simulink model "SVPWMtrialsweird"  (R2015b)
settings: Solver=VariableStepAuto  StartTime=0.0  StopTime=0.05  RelTol=1e-3
libraries: powerlib x29, simulink x1
(part 2 of 2)

== matlab function SVPWMtrialsweird/sequencing ==
  data: a input; rgn2a input; rgn2b input; rgn3 input; rgn4 input; Sector1 input; Sector2 input; Sector3 input; Sector4 input; Sector5 input; Sector6 input; Ta input; Tb input; Tc input; Sa1 output; Sa2 output; Sa1P output; Sa2P output; time input; Sb1 output; Sb2 output; Sb1P output; Sb2P output; Sc1 output; Sc2 output; Sc1P output; Sc2P output; exttime input
function [Sa1, Sa2, Sa1P, Sa2P, Sb1, Sb2, Sb1P, Sb2P, Sc1, Sc2, Sc1P, Sc2P] = fcn(a,rgn2a,rgn2b,rgn3,rgn4,Sector1,Sector2, Sector3, Sector4, Sector5,Sector6,Ta, Tb, Tc, time,exttime)
% this program works for magnitude of Vref is greater then Vd/3 meaning ma
% must be greater than 1/sqrt(3). for smaller ma's computation is a bit
% more tricky therefore it is omitted for simplicity for now. 
% % Vref = ma*Vd/sqrt(3); %magnitude of Vref
% % theta = 2*pi*fundf*time; %angle of Vref
% % angle = mod(theta, 2*pi);
% % Ts = 1/swf;
% % Ta = 0;
% % Tb = 0;
% % Tc = 0;
% % output = 0;
% % Sector1 = 0; Sector2 = 0; Sector3 = 0; Sector4= 0; Sector5 = 0; Sector6 = 0;
% % rgn2 = 0 ; rgn3 = 0; rgn4 = 0;
Sa1=0; Sa2=0; Sa1P=0; Sa2P=0; Sb1=0; Sb2=0; Sb1P=0; Sb2P=0; Sc1=0; Sc2=0; Sc1P=0; Sc2P=0;
%a = exttime;
%% Sequencing Part
if(Sector1)
    if(rgn3)
        while(a<exttime+Tc/4)
            Sa1=0; Sa2=1; Sa1P=1; Sa2P=0;
            Sb1=0; Sb2=0; Sb1P=1; Sb2P=1; 
            Sc1=0; Sc2=0; Sc1P=1; Sc2P=1;
            a = a+0.000001; %pause(Tc/4); 
        end
        while(a<exttime+Tb/2)
            Sa1=1; Sa2=1; Sa1P=0; Sa2P=0;
            Sb1=0; Sb2=0; Sb1P=1; Sb2P=1; 
            Sc1=0; Sc2=0; Sc1P=1; Sc2P=1;
            a = a+0.000001;%pause(Tb/2);
        end
        while(a<exttime+Ta/2)
            Sa1=1; Sa2=1; Sa1P=0; Sa2P=0;
            Sb1=0; Sb2=1; Sb1P=1; Sb2P=0; 
            Sc1=0; Sc2=0; Sc1P=1; Sc2P=1;
            a = a+0.000001; %pause(Ta/2); 
        end
        while(a<exttime+Tc/2)
            Sa1=1; Sa2=1; Sa1P=0; Sa2P=0;
            Sb1=0; Sb2=1; Sb1P=1; Sb2P=0; 
            Sc1=0; Sc2=1; Sc1P=1; Sc2P=0;
            a = a+0.000001; %pause(Tc/2);
        end
        while(a<exttime+Ta/2)
            Sa1=1; Sa2=1; Sa1P=0; Sa2P=0;
            Sb1=0; Sb2=1; Sb1P=1; Sb2P=0; 
            Sc1=0; Sc2=0; Sc1P=1; Sc2P=1;
            a = a+0.000001; %pause(Ta/2); 
        end
        while(a<exttime+Tb/2)
            Sa1=1; Sa2=1; Sa1P=0; Sa2P=0;
            Sb1=0; Sb2=0; Sb1P=1; Sb2P=1; 
            Sc1=0; Sc2=0; Sc1P=1; Sc2P=1;
            a = a+0.000001; %pause(Tb/2); 
        end
        while(a<exttime+Tc/4)
            Sa1=0; Sa2=1; Sa1P=1; Sa2P=0;
            Sb1=0; Sb2=0; Sb1P=1; Sb2P=1; 
            Sc1=0; Sc2=0; Sc1P=1; Sc2P=1;
            a = a+0.000001; %pause(Tc/4);        
        end
    end

        if(rgn2a)
            while(a<exttime+Tc/4)
                Sa1=0; Sa2=1; Sa1P=1; Sa2P=0;
                Sb1=0; Sb2=0; Sb1P=1; Sb2P=1; 
                Sc1=0; Sc2=0; Sc1P=1; Sc2P=1;
            a = a+0.000001; %pause(Tc/4);
            end
            while(a<exttime+Tb/2)
                Sa1=0; Sa2=1; Sa1P=1; Sa2P=0;
                Sb1=0; Sb2=1; Sb1P=1; Sb2P=0; 
                Sc1=0; Sc2=0; Sc1P=1; Sc2P=1;
                a = a+0.000001; %pause(Tb/2); 
            end
            while(a<exttime+Ta/2)
                Sa1=1; Sa2=1; Sa1P=0; Sa2P=0;
                Sb1=0; Sb2=1; Sb1P=1; Sb2P=0; 
                Sc1=0; Sc2=0; Sc1P=1; Sc2P=1;       
                a = a+0.000001; %pause(Ta/2); 
            end
            while(a<exttime+Tc/2)
                Sa1=1; Sa2=1; Sa1P=0; Sa2P=0;
                Sb1=0; Sb2=1; Sb1P=1; Sb2P=0; 
                Sc1=0; Sc2=1; Sc1P=1; Sc2P=0;
            a = a+0.000001; %pause(Tc/2);
            end
            while(a<exttime+Ta/2)
                Sa1=1; Sa2=1; Sa1P=0; Sa2P=0;
                Sb1=0; Sb2=1; Sb1P=1; Sb2P=0; 
                Sc1=0; Sc2=0; Sc1P=1; Sc2P=1;
                a = a+0.000001; %pause(Ta/2); 
            end
            while(a<exttime+Tb/2)
                Sa1=0; Sa2=1; Sa1P=1; Sa2P=0;
                Sb1=0; Sb2=1; Sb1P=1; Sb2P=0; 
                Sc1=0; Sc2=0; Sc1P=1; Sc2P=1;
                a = a+0.000001; %pause(Tb/2); 
            end
            while(a<exttime+Tc/4)
                Sa1=0; Sa2=1; Sa1P=1; Sa2P=0;
                Sb1=0; Sb2=0; Sb1P=1; Sb2P=1; 
                Sc1=0; Sc2=0; Sc1P=1; Sc2P=1;
                a = a+0.000001; %pause(Tc/4);        
            end
        end
        if(rgn2b)
            while(a<exttime+Tc/4)
                Sa1=0; Sa2=1; Sa1P=1; Sa2P=0;
                Sb1=0; Sb2=1; Sb1P=1; Sb2P=0; 
                Sc1=0; Sc2=0; Sc1P=1; Sc2P=1;
                a = a+0.000001; %pause(Tc/4);
            end
            while(a<exttime+Tb/2)
                Sa1=1; Sa2=1; Sa1P=0; Sa2P=0;
                Sb1=0; Sb2=1; Sb1P=1; Sb2P=0; 
                Sc1=0; Sc2=0; Sc1P=1; Sc2P=1;
                a = a+0.000001; %pause(Tb/2); 
            end
            while(a<exttime+Ta/2)
                Sa1=1; Sa2=1; Sa1P=0; Sa2P=0;
                Sb1=0; Sb2=1; Sb1P=1; Sb2P=0; 
                Sc1=0; Sc2=1; Sc1P=1; Sc2P=0;
                a = a+0.000001; %pause(Ta/2); 
            end
            while(a<exttime+Tc/2)
                Sa1=1; Sa2=1; Sa1P=0; Sa2P=0;
                Sb1=1; Sb2=1; Sb1P=0; Sb2P=0; 
                Sc1=0; Sc2=1; Sc1P=1; Sc2P=0;
                a = a+0.000001; %pause(Tc/2);
            end
            while(a<exttime+Ta/2)
                Sa1=1; Sa2=1; Sa1P=0; Sa2P=0;
                Sb1=0; Sb2=1; Sb1P=1; Sb2P=0; 
                Sc1=0; Sc2=1; Sc1P=1; Sc2P=0;
                a = a+0.000001; %pause(Ta/2); 
            end
            while(a<exttime+Tb/2)
                Sa1=1; Sa2=1; Sa1P=0; Sa2P=0;
                Sb1=0; Sb2=1; Sb1P=1; Sb2P=0; 
                Sc1=0; Sc2=0; Sc1P=1; Sc2P=1;
                a = a+0.000001; %pause(Tb/2); 
            end
            while(a<exttime+Tc/4)
                Sa1=0; Sa2=1; Sa1P=1; Sa2P=0;
                Sb1=0; Sb2=1; Sb1P=1; Sb2P=0; 
                Sc1=0; Sc2=0; Sc1P=1; Sc2P=1;
                a = a+0.000001; %pause(Tc/4);
            end
        end
    if(rgn4)
        while(a<exttime+Tc/4)
            Sa1=0; Sa2=1; Sa1P=1; Sa2P=0;
            Sb1=0; Sb2=1; Sb1P=1; Sb2P=0;
            Sc1=0; Sc2=0; Sc1P=1; Sc2P=1;
            a = a+0.000001; %pause(Tc/4);
        end
        while(a<exttime+Tb/2)
            Sa1=1; Sa2=1; Sa1P=0; Sa2P=0;
            Sb1=0; Sb2=1; Sb1P=1; Sb2P=0;
            Sc1=0; Sc2=0; Sc1P=1; Sc2P=1;        
            a = a+0.000001; %pause(Tb/2);         
        end
        while(a<exttime+Ta/2)
            Sa1=1; Sa2=1; Sa1P=0; Sa2P=0;
            Sb1=1; Sb2=1; Sb1P=0; Sb2P=0;
            Sc1=0; Sc2=0; Sc1P=1; Sc2P=1;
            a = a+0.000001; %pause(Ta/2); 
        end
        while(a<exttime+Tc/2)
            Sa1=1; Sa2=1; Sa1P=0; Sa2P=0;
            Sb1=1; Sb2=1; Sb1P=0; Sb2P=0;
            Sc1=0; Sc2=1; Sc1P=1; Sc2P=0;
            a = a+0.000001; %pause(Tc/2);
        end
        while(a<exttime+Ta/2)
            Sa1=1; Sa2=1; Sa1P=0; Sa2P=0;
            Sb1=1; Sb2=1; Sb1P=0; Sb2P=0;
            Sc1=0; Sc2=0; Sc1P=1; Sc2P=1;
            a = a+0.000001; %pause(Ta/2);         
        end
        while(a<exttime+Tb/2)
            Sa1=1; Sa2=1; Sa1P=0; Sa2P=0;
            Sb1=0; Sb2=1; Sb1P=1; Sb2P=0;
            Sc1=0; Sc2=0; Sc1P=1; Sc2P=1;        
            a = a+0.000001; %pause(Tb/2); 
        end
        while(a<exttime+Tc/4)
            Sa1=0; Sa2=1; Sa1P=1; Sa2P=0;
            Sb1=0; Sb2=1; Sb1P=1; Sb2P=0;
            Sc1=0; Sc2=0; Sc1P=1; Sc2P=1;
            a = a+0.000001; %pause(Tc/4);
        end
    end
end
if(Sector2)
    if(rgn3)
        while(a<exttime+Tc/4)
            Sa1=0; Sa2=1; Sa1P=1; Sa2P=0;
            Sb1=0; Sb2=1; Sb1P=1; Sb2P=0;
            Sc1=0; Sc2=0; Sc1P=1; Sc2P=1;
        a = a+0.000001; %pause(Tc/4);
        end
        while(a<exttime+Tb/2)
            Sa1=0; Sa2=1; Sa1P=1; Sa2P=0;
            Sb1=1; Sb2=1; Sb1P=0; Sb2P=0;
            Sc1=0; Sc2=0; Sc1P=1; Sc2P=1;
            a = a+0.000001; %pause(Tb/2); 
        end
        while(a<exttime+Ta/2)
            Sa1=1; Sa2=1; Sa1P=0; Sa2P=0;
            Sb1=1; Sb2=1; Sb1P=0; Sb2P=0;
            Sc1=0; Sc2=0; Sc1P=1; Sc2P=1;
            a = a+0.000001; %pause(Ta/2); 
        end
        while(a<exttime+Tc/2)
            Sa1=1; Sa2=1; Sa1P=0; Sa2P=0;
            Sb1=1; Sb2=1; Sb1P=0; Sb2P=0;
            Sc1=0; Sc2=1; Sc1P=1; Sc2P=0;       
            a = a+0.000001; %pause(Tc/2);
        end
        while(a<exttime+Ta/2)
            Sa1=1; Sa2=1; Sa1P=0; Sa2P=0;
            Sb1=1; Sb2=1; Sb1P=0; Sb2P=0;
            Sc1=0; Sc2=0; Sc1P=1; Sc2P=1;
            a = a+0.000001; %pause(Ta/2); 
        end
        while(a<exttime+Tb/2)
            Sa1=0; Sa2=1; Sa1P=1; Sa2P=0;
            Sb1=1; Sb2=1; Sb1P=0; Sb2P=0;
            Sc1=0; Sc2=0; Sc1P=1; Sc2P=1;
            a = a+0.000001; %pause(Tb/2); 
        end
        while(a<exttime+Tc/4)
            Sa1=0; Sa2=1; Sa1P=1; Sa2P=0;
            Sb1=0; Sb2=1; Sb1P=1; Sb2P=0;
            Sc1=0; Sc2=0; Sc1P=1; Sc2P=1;
            a = a+0.000001; %pause(Tc/4);       
        end
    end
    
        if(rgn2a)
            while(a<exttime+Tc/4)
                Sa1=0; Sa2=1; Sa1P=1; Sa2P=0;
                Sb1=0; Sb2=1; Sb1P=1; Sb2P=0;
                Sc1=0; Sc2=0; Sc1P=1; Sc2P=1;
                a = a+0.000001; %pause(Tc/4);
            end
            while(a<exttime+Tb/2)
                Sa1=0; Sa2=1; Sa1P=1; Sa2P=0;
                Sb1=1; Sb2=1; Sb1P=0; Sb2P=0;
                Sc1=0; Sc2=0; Sc1P=1; Sc2P=1;
                a = a+0.000001; %pause(Tb/2); 
            end
            while(a<exttime+Ta/2)
                Sa1=0; Sa2=1; Sa1P=1; Sa2P=0;
                Sb1=1; Sb2=1; Sb1P=0; Sb2P=0;
                Sc1=0; Sc2=1; Sc1P=1; Sc2P=0;
                a = a+0.000001; %pause(Ta/2); 
            end
            while(a<exttime+Tc/2)
                Sa1=1; Sa2=1; Sa1P=0; Sa2P=0;
                Sb1=1; Sb2=1; Sb1P=0; Sb2P=0;
                Sc1=0; Sc2=1; Sc1P=1; Sc2P=0;            
                a = a+0.000001; %pause(Tc/2);
            end
            while(a<exttime+Ta/2)
                Sa1=0; Sa2=1; Sa1P=1; Sa2P=0;
                Sb1=1; Sb2=1; Sb1P=0; Sb2P=0;
                Sc1=0; Sc2=1; Sc1P=1; Sc2P=0;
                a = a+0.000001; %pause(Ta/2); 
            end
            while(a<exttime+Tb/2)
                Sa1=0; Sa2=1; Sa1P=1; Sa2P=0;
                Sb1=1; Sb2=1; Sb1P=0; Sb2P=0;
                Sc1=0; Sc2=0; Sc1P=1; Sc2P=1;
                a = a+0.000001; %pause(Tb/2); 
            end
            while(a<exttime+Tc/4)
                Sa1=0; Sa2=1; Sa1P=1; Sa2P=0;
                Sb1=0; Sb2=1; Sb1P=1; Sb2P=0;
                Sc1=0; Sc2=0; Sc1P=1; Sc2P=1;
                a = a+0.000001; %pause(Tc/4);
            end
        end
        if(rgn2b)
            while(a<exttime+Tc/4)
                Sa1=0; Sa2=0; Sa1P=1; Sa2P=1;
                Sb1=0; Sb2=1; Sb1P=1; Sb2P=0;
                Sc1=0; Sc2=0; Sc1P=1; Sc2P=1;
                a = a+0.000001; %pause(Tc/4);
            end
            while(a<exttime+Tb/2)
                Sa1=0; Sa2=1; Sa1P=1; Sa2P=0;
                Sb1=0; Sb2=1; Sb1P=1; Sb2P=0;
                Sc1=0; Sc2=0; Sc1P=1; Sc2P=1;
                a = a+0.000001; %pause(Tb/2); 
            end
            while(a<exttime+Ta/2)
                Sa1=0; Sa2=1; Sa1P=1; Sa2P=0;
                Sb1=1; Sb2=1; Sb1P=0; Sb2P=0;
                Sc1=0; Sc2=0; Sc1P=1; Sc2P=1;
                a = a+0.000001; %pause(Ta/2); 
            end
            while(a<exttime+Tc/2)
                Sa1=0; Sa2=1; Sa1P=1; Sa2P=0;   
                Sb1=1; Sb2=1; Sb1P=0; Sb2P=0;
                Sc1=0; Sc2=1; Sc1P=1; Sc2P=0;
                a = a+0.000001; %pause(Tc/2);
            end
            while(a<exttime+Ta/2)
                Sa1=0; Sa2=1; Sa1P=1; Sa2P=0;
                Sb1=1; Sb2=1; Sb1P=0; Sb2P=0;
                Sc1=0; Sc2=0; Sc1P=1; Sc2P=1;
                a = a+0.000001; %pause(Ta/2); 
            end
            while(a<exttime+Tb/2)
                Sa1=0; Sa2=1; Sa1P=1; Sa2P=0;
                Sb1=0; Sb2=1; Sb1P=1; Sb2P=0;
                Sc1=0; Sc2=0; Sc1P=1; Sc2P=1;
                a = a+0.000001; %pause(Tb/2); 
            end
            while(a<exttime+Tc/4)
                Sa1=0; Sa2=0; Sa1P=1; Sa2P=1;
                Sb1=0; Sb2=1; Sb1P=1; Sb2P=0;
                Sc1=0; Sc2=0; Sc1P=1; Sc2P=1;
                a = a+0.000001; %pause(Tc/4);           
            end
        end    
    if(rgn4)
        while(a<exttime+Tc/4)
            Sa1=0; Sa2=0; Sa1P=1; Sa2P=1;
            Sb1=0; Sb2=1; Sb1P=1; Sb2P=0;
            Sc1=0; Sc2=0; Sc1P=1; Sc2P=1;
            a = a+0.000001; %pause(Tc/4);
        end
        while(a<exttime+Tb/2)
            Sa1=0; Sa2=0; Sa1P=1; Sa2P=1;
            Sb1=1; Sb2=1; Sb1P=0; Sb2P=0;
            Sc1=0; Sc2=0; Sc1P=1; Sc2P=1;
            a = a+0.000001; %pause(Tb/2); 
        end
        while(a<exttime+Ta/2)
            Sa1=0; Sa2=1; Sa1P=1; Sa2P=0;
            Sb1=1; Sb2=1; Sb1P=0; Sb2P=0;
            Sc1=0; Sc2=0; Sc1P=1; Sc2P=1;
            a = a+0.000001; %pause(Ta/2); 
        end
        while(a<exttime+Tc/2)
            Sa1=0; Sa2=1; Sa1P=1; Sa2P=0;
            Sb1=1; Sb2=1; Sb1P=0; Sb2P=0;
            Sc1=0; Sc2=1; Sc1P=1; Sc2P=0;
            a = a+0.000001; %pause(Tc/2); 
        end
        while(a<exttime+Ta/2)
            Sa1=0; Sa2=1; Sa1P=1; Sa2P=0;
            Sb1=1; Sb2=1; Sb1P=0; Sb2P=0;
            Sc1=0; Sc2=0; Sc1P=1; Sc2P=1;
            a = a+0.000001; %pause(Ta/2); 
        end
        while(a<exttime+Tb/2)
            Sa1=0; Sa2=0; Sa1P=1; Sa2P=1;
            Sb1=1; Sb2=1; Sb1P=0; Sb2P=0;
            Sc1=0; Sc2=0; Sc1P=1; Sc2P=1;
            a = a+0.000001; %pause(Tb/2); 
        end
        while(a<exttime+Tc/4)
            Sa1=0; Sa2=0; Sa1P=1; Sa2P=1;
            Sb1=0; Sb2=1; Sb1P=1; Sb2P=0;
            Sc1=0; Sc2=0; Sc1P=1; Sc2P=1;
            a = a+0.000001; %pause(Tc/4);
        end
    end

end
if(Sector3)
    if(rgn3)
        while(a<exttime+Tc/4)
            Sa1=0; Sa2=0; Sa1P=1; Sa2P=1;
            Sb1=0; Sb2=1; Sb1P=1; Sb2P=0;
            Sc1=0; Sc2=0; Sc1P=1; Sc2P=1;
            a = a+0.000001; %pause(Tc/4);
        end
        while(a<exttime+Tb/2)
            Sa1=0; Sa2=0; Sa1P=1; Sa2P=1;
            Sb1=1; Sb2=1; Sb1P=0; Sb2P=0;
            Sc1=0; Sc2=0; Sc1P=1; Sc2P=1;
            a = a+0.000001; %pause(Tb/2); 
        end
        while(a<exttime+Ta/2)
            Sa1=0; Sa2=0; Sa1P=1; Sa2P=1;
            Sb1=1; Sb2=1; Sb1P=0; Sb2P=0;
            Sc1=0; Sc2=1; Sc1P=1; Sc2P=0;
            a = a+0.000001; %pause(Ta/2); 
        end
        while(a<exttime+Tc/2)
            Sa1=0; Sa2=1; Sa1P=1; Sa2P=0;
            Sb1=1; Sb2=1; Sb1P=0; Sb2P=0;
            Sc1=0; Sc2=1; Sc1P=1; Sc2P=0;
            a = a+0.000001; %pause(Tc/2);
        end
        while(a<exttime+Ta/2)
            Sa1=0; Sa2=0; Sa1P=1; Sa2P=1;
            Sb1=1; Sb2=1; Sb1P=0; Sb2P=0;
            Sc1=0; Sc2=1; Sc1P=1; Sc2P=0;
            a = a+0.000001; %pause(Ta/2); 
        end
        while(a<exttime+Tb/2)
            Sa1=0; Sa2=0; Sa1P=1; Sa2P=1;
            Sb1=1; Sb2=1; Sb1P=0; Sb2P=0;
            Sc1=0; Sc2=0; Sc1P=1; Sc2P=1;
            a = a+0.000001; %pause(Tb/2); 
        end
        while(a<exttime+Tc/4)
            Sa1=0; Sa2=0; Sa1P=1; Sa2P=1;
            Sb1=0; Sb2=1; Sb1P=1; Sb2P=0;
            Sc1=0; Sc2=0; Sc1P=1; Sc2P=1;
            a = a+0.000001; %pause(Tc/4);        
        end
    end

        if(rgn2a)
            while(a<exttime+Tc/4)            
                Sa1=0; Sa2=0; Sa1P=1; Sa2P=1;
                Sb1=0; Sb2=1; Sb1P=1; Sb2P=0;
                Sc1=0; Sc2=0; Sc1P=1; Sc2P=1;
                a = a+0.000001; %pause(Tc/4);
            end
            while(a<exttime+Tb/2)
                Sa1=0; Sa2=0; Sa1P=1; Sa2P=1;
                Sb1=0; Sb2=1; Sb1P=1; Sb2P=0;
                Sc1=0; Sc2=1; Sc1P=1; Sc2P=0;
                a = a+0.000001; %pause(Tb/2); 
            end
            while(a<exttime+Ta/2)
                Sa1=0; Sa2=0; Sa1P=1; Sa2P=1;
                Sb1=1; Sb2=1; Sb1P=0; Sb2P=0;
                Sc1=0; Sc2=1; Sc1P=1; Sc2P=0;
            	a = a+0.000001; %pause(Ta/2); 
            end
            while(a<exttime+Tc/2)
                Sa1=0; Sa2=0; Sa1P=1; Sa2P=1;
                Sb1=1; Sb2=1; Sb1P=0; Sb2P=0;
                Sc1=0; Sc2=0; Sc1P=1; Sc2P=1;
                a = a+0.000001; %pause(Tc/2);
            end
            while(a<exttime+Ta/2)
                Sa1=0; Sa2=0; Sa1P=1; Sa2P=1;
                Sb1=1; Sb2=1; Sb1P=0; Sb2P=0;
                Sc1=0; Sc2=1; Sc1P=1; Sc2P=0;
                a = a+0.000001; %pause(Ta/2); 
            end
            while(a<exttime+Tb/2)
                Sa1=0; Sa2=0; Sa1P=1; Sa2P=1;
                Sb1=0; Sb2=1; Sb1P=1; Sb2P=0;
                Sc1=0; Sc2=1; Sc1P=1; Sc2P=0;
                a = a+0.000001; %pause(Tb/2); 
            end
            while(a<exttime+Tc/4)
                Sa1=0; Sa2=0; Sa1P=1; Sa2P=1;
                Sb1=0; Sb2=1; Sb1P=1; Sb2P=0;
                Sc1=0; Sc2=0; Sc1P=1; Sc2P=1;
                a = a+0.000001; %pause(Tc/4); 
            end
        end
        if(rgn2b)
            while(a<exttime+Tc/4)
                Sa1=0; Sa2=0; Sa1P=1; Sa2P=1;
                Sb1=0; Sb2=1; Sb1P=1; Sb2P=0;
                Sc1=0; Sc2=1; Sc1P=1; Sc2P=0;
                a = a+0.000001; %pause(Tc/4);
            end
            while(a<exttime+Tb/2)
                Sa1=0; Sa2=0; Sa1P=1; Sa2P=1;
                Sb1=1; Sb2=1; Sb1P=0; Sb2P=0;
                Sc1=0; Sc2=1; Sc1P=1; Sc2P=0;
                a = a+0.000001; %pause(Tb/2); 
            end
            while(a<exttime+Ta/2)
                Sa1=0; Sa2=1; Sa1P=1; Sa2P=0;
                Sb1=1; Sb2=1; Sb1P=0; Sb2P=0;
                Sc1=0; Sc2=1; Sc1P=1; Sc2P=0;
                a = a+0.000001; %pause(Ta/2); 
            end
            while(a<exttime+Tc/2)
                Sa1=0; Sa2=1; Sa1P=1; Sa2P=0;
                Sb1=1; Sb2=1; Sb1P=0; Sb2P=0;
                Sc1=1; Sc2=1; Sc1P=0; Sc2P=0;
                a = a+0.000001; %pause(Tc/2);
            end
            while(a<exttime+Ta/2)
                Sa1=0; Sa2=1; Sa1P=1; Sa2P=0;
                Sb1=1; Sb2=1; Sb1P=0; Sb2P=0;
                Sc1=0; Sc2=1; Sc1P=1; Sc2P=0;
                a = a+0.000001; %pause(Ta/2); 
            end
            while(a<exttime+Tb/2)
                Sa1=0; Sa2=0; Sa1P=1; Sa2P=1;
                Sb1=1; Sb2=1; Sb1P=0; Sb2P=0;
                Sc1=0; Sc2=1; Sc1P=1; Sc2P=0;
                a = a+0.000001; %pause(Tb/2); 
            end
            while(a<exttime+Tc/4)
                Sa1=0; Sa2=0; Sa1P=1; Sa2P=1;
                Sb1=0; Sb2=1; Sb1P=1; Sb2P=0;
                Sc1=0; Sc2=1; Sc1P=1; Sc2P=0;
                a = a+0.000001; %pause(Tc/4);            
            end
        end

    if(rgn4)
        while(a<exttime+Tc/4)
            Sa1=0; Sa2=0; Sa1P=1; Sa2P=1;
            Sb1=0; Sb2=1; Sb1P=1; Sb2P=0;
            Sc1=0; Sc2=1; Sc1P=1; Sc2P=0;
            a = a+0.000001; %pause(Tc/4);
        end
        while(a<exttime+Tb/2)
            Sa1=0; Sa2=0; Sa1P=1; Sa2P=1;
            Sb1=1; Sb2=1; Sb1P=0; Sb2P=0;
            Sc1=0; Sc2=1; Sc1P=1; Sc2P=0;
            a = a+0.000001; %pause(Tb/2); 
        end
        while(a<exttime+Ta/2)
            Sa1=0; Sa2=0; Sa1P=1; Sa2P=1;
            Sb1=1; Sb2=1; Sb1P=0; Sb2P=0;
            Sc1=1; Sc2=1; Sc1P=0; Sc2P=0;
            a = a+0.000001; %pause(Ta/2); 
        end
        while(a<exttime+Tc/2)
            Sa1=0; Sa2=1; Sa1P=1; Sa2P=0;
            Sb1=1; Sb2=1; Sb1P=0; Sb2P=0;
            Sc1=1; Sc2=1; Sc1P=0; Sc2P=0;
            a = a+0.000001; %pause(Tc/2);
        end
        while(a<exttime+Ta/2)
            Sa1=0; Sa2=0; Sa1P=1; Sa2P=1;
            Sb1=1; Sb2=1; Sb1P=0; Sb2P=0;
            Sc1=1; Sc2=1; Sc1P=0; Sc2P=0;
            a = a+0.000001; %pause(Ta/2); 
        end
        while(a<exttime+Tb/2)
            Sa1=0; Sa2=0; Sa1P=1; Sa2P=1;
            Sb1=1; Sb2=1; Sb1P=0; Sb2P=0;
            Sc1=0; Sc2=1; Sc1P=1; Sc2P=0;
            a = a+0.000001; %pause(Tb/2); 
        end
        while(a<exttime+Tc/4)
            Sa1=0; Sa2=0; Sa1P=1; Sa2P=1;
            Sb1=0; Sb2=1; Sb1P=1; Sb2P=0;
            Sc1=0; Sc2=1; Sc1P=1; Sc2P=0;
            a = a+0.000001; %pause(Tc/4);
        end
    end
end
if(Sector4)
    if(rgn3) 
        while(a<exttime+Tc/4)
            Sa1=0; Sa2=1; Sa1P=1; Sa2P=0;
            Sb1=1; Sb2=1; Sb1P=0; Sb2P=0;
            Sc1=1; Sc2=1; Sc1P=0; Sc2P=0;
            a = a+0.000001; %pause(Tc/4);
        end
        while(a<exttime+Tb/2)
            Sa1=0; Sa2=0; Sa1P=1; Sa2P=1;
            Sb1=1; Sb2=1; Sb1P=0; Sb2P=0;
            Sc1=1; Sc2=1; Sc1P=0; Sc2P=0;
            a = a+0.000001; %pause(Tb/2); 
        end
        while(a<exttime+Ta/2)
            Sa1=0; Sa2=0; Sa1P=1; Sa2P=1;
            Sb1=0; Sb2=1; Sb1P=1; Sb2P=0;
            Sc1=1; Sc2=1; Sc1P=0; Sc2P=0;
            a = a+0.000001; %pause(Ta/2); 
        end
        while(a<exttime+Tc/2)
            Sa1=0; Sa2=0; Sa1P=1; Sa2P=1;
            Sb1=0; Sb2=1; Sb1P=1; Sb2P=0;
            Sc1=0; Sc2=1; Sc1P=1; Sc2P=0;
            a = a+0.000001; %pause(Tc/2);
        end
        while(a<exttime+Ta/2)
            Sa1=0; Sa2=0; Sa1P=1; Sa2P=1;
            Sb1=0; Sb2=1; Sb1P=1; Sb2P=0;
            Sc1=1; Sc2=1; Sc1P=0; Sc2P=0;
            a = a+0.000001; %pause(Ta/2); 
        end
        while(a<exttime+Tb/2)
            Sa1=0; Sa2=0; Sa1P=1; Sa2P=1;
            Sb1=1; Sb2=1; Sb1P=0; Sb2P=0;
            Sc1=1; Sc2=1; Sc1P=0; Sc2P=0;
            a = a+0.000001; %pause(Tb/2); 
        end
        while(a<exttime+Tc/4)
            Sa1=0; Sa2=1; Sa1P=1; Sa2P=0;
            Sb1=1; Sb2=1; Sb1P=0; Sb2P=0;
            Sc1=1; Sc2=1; Sc1P=0; Sc2P=0;
            a = a+0.000001; %pause(Tc/4);
        end
    end
        if(rgn2a)
            while(a<exttime+Tc/4)
                Sa1=0; Sa2=1; Sa1P=1; Sa2P=0;
                Sb1=1; Sb2=1; Sb1P=0; Sb2P=0;
                Sc1=1; Sc2=1; Sc1P=0; Sc2P=0;
                a = a+0.000001; %pause(Tc/4);
            end
            while(a<exttime+Tb/2)
                Sa1=0; Sa2=1; Sa1P=1; Sa2P=0;
                Sb1=0; Sb2=1; Sb1P=1; Sb2P=0;
                Sc1=1; Sc2=1; Sc1P=0; Sc2P=0;
                a = a+0.000001; %pause(Tb/2); 
            end
            while(a<exttime+Ta/2)
                Sa1=0; Sa2=0; Sa1P=1; Sa2P=1;
                Sb1=0; Sb2=1; Sb1P=1; Sb2P=0;
                Sc1=1; Sc2=1; Sc1P=0; Sc2P=0;
                a = a+0.000001; %pause(Ta/2); 
            end
            while(a<exttime+Tc/2)
                Sa1=0; Sa2=0; Sa1P=1; Sa2P=1;
                Sb1=0; Sb2=1; Sb1P=1; Sb2P=0;
                Sc1=0; Sc2=1; Sc1P=1; Sc2P=0;
                a = a+0.000001; %pause(Tc/2);
            end
            while(a<exttime+Ta/2)
                Sa1=0; Sa2=0; Sa1P=1; Sa2P=1;
                Sb1=0; Sb2=1; Sb1P=1; Sb2P=0;
                Sc1=1; Sc2=1; Sc1P=0; Sc2P=0;
                a = a+0.000001; %pause(Ta/2); 
            end
            while(a<exttime+Tb/2)
                Sa1=0; Sa2=1; Sa1P=1; Sa2P=0;
                Sb1=0; Sb2=1; Sb1P=1; Sb2P=0;
                Sc1=1; Sc2=1; Sc1P=0; Sc2P=0;
                a = a+0.000001; %pause(Tb/2); 
            end
            while(a<exttime+Tc/4)
                Sa1=0; Sa2=1; Sa1P=1; Sa2P=0;
                Sb1=1; Sb2=1; Sb1P=0; Sb2P=0;
                Sc1=1; Sc2=1; Sc1P=0; Sc2P=0;
                a = a+0.000001; %pause(Tc/4);           
            end
        end
        if(rgn2b)
            while(a<exttime+Tc/4)
                Sa1=0; Sa2=1; Sa1P=1; Sa2P=0;
                Sb1=0; Sb2=1; Sb1P=1; Sb2P=0;
                Sc1=1; Sc2=1; Sc1P=0; Sc2P=0;
                a = a+0.000001; %pause(Tc/4);
            end
            while(a<exttime+Tb/2)
                Sa1=0; Sa2=0; Sa1P=1; Sa2P=1;
                Sb1=0; Sb2=1; Sb1P=1; Sb2P=0;
                Sc1=1; Sc2=1; Sc1P=0; Sc2P=0;
            a = a+0.000001; %pause(Tb/2); 
            end
            while(a<exttime+Ta/2)
                Sa1=0; Sa2=0; Sa1P=1; Sa2P=1;
                Sb1=0; Sb2=1; Sb1P=1; Sb2P=0;
                Sc1=0; Sc2=1; Sc1P=1; Sc2P=0;
                a = a+0.000001; %pause(Ta/2); 
            end
            while(a<exttime+Tc/2)
                Sa1=0; Sa2=0; Sa1P=1; Sa2P=1;
                Sb1=0; Sb2=0; Sb1P=1; Sb2P=1;
                Sc1=0; Sc2=1; Sc1P=1; Sc2P=0;
                a = a+0.000001; %pause(Tc/2);
            end
            while(a<exttime+Ta/2)
                Sa1=0; Sa2=0; Sa1P=1; Sa2P=1;
                Sb1=0; Sb2=1; Sb1P=1; Sb2P=0;
                Sc1=0; Sc2=1; Sc1P=1; Sc2P=0;
                a = a+0.000001; %pause(Ta/2); 
            end
            while(a<exttime+Tb/2)
                Sa1=0; Sa2=0; Sa1P=1; Sa2P=1;
                Sb1=0; Sb2=1; Sb1P=1; Sb2P=0;
                Sc1=1; Sc2=1; Sc1P=0; Sc2P=0;
                a = a+0.000001; %pause(Tb/2); 
            end
            while(a<exttime+Tc/4)
                Sa1=0; Sa2=1; Sa1P=1; Sa2P=0;
                Sb1=0; Sb2=1; Sb1P=1; Sb2P=0;
                Sc1=1; Sc2=1; Sc1P=0; Sc2P=0;
                a = a+0.000001; %pause(Tc/4);                      
            end
        end
    if(rgn4)
        while(a<exttime+Tc/4)
            Sa1=0; Sa2=1; Sa1P=1; Sa2P=0;
            Sb1=0; Sb2=1; Sb1P=1; Sb2P=0;
            Sc1=1; Sc2=1; Sc1P=0; Sc2P=0;
            a = a+0.000001; %pause(Tc/4);
        end
        while(a<exttime+Tb/2)
            Sa1=0; Sa2=0; Sa1P=1; Sa2P=1;
            Sb1=0; Sb2=1; Sb1P=1; Sb2P=0;
            Sc1=1; Sc2=1; Sc1P=0; Sc2P=0;
            a = a+0.000001; %pause(Tb/2); 
        end
        while(a<exttime+Ta/2)
            Sa1=0; Sa2=0; Sa1P=1; Sa2P=1;
            Sb1=0; Sb2=0; Sb1P=1; Sb2P=1;
            Sc1=1; Sc2=1; Sc1P=0; Sc2P=0;
            a = a+0.000001; %pause(Ta/2); 
        end
        while(a<exttime+Tc/2)
            Sa1=0; Sa2=0; Sa1P=1; Sa2P=1;
            Sb1=0; Sb2=0; Sb1P=1; Sb2P=1;
            Sc1=0; Sc2=1; Sc1P=1; Sc2P=0;
            a = a+0.000001; %pause(Tc/2);
        end
        while(a<exttime+Ta/2)
            Sa1=0; Sa2=0; Sa1P=1; Sa2P=1;
            Sb1=0; Sb2=0; Sb1P=1; Sb2P=1;
            Sc1=1; Sc2=1; Sc1P=0; Sc2P=0;
            a = a+0.000001; %pause(Ta/2); 
        end
        while(a<exttime+Tb/2)
            Sa1=0; Sa2=0; Sa1P=1; Sa2P=1;
            Sb1=0; Sb2=1; Sb1P=1; Sb2P=0;
            Sc1=1; Sc2=1; Sc1P=0; Sc2P=0;
            a = a+0.000001; %pause(Tb/2); 
        end
        while(a<exttime+Tc/4)
            Sa1=0; Sa2=1; Sa1P=1; Sa2P=0;
            Sb1=0; Sb2=1; Sb1P=1; Sb2P=0;
            Sc1=1; Sc2=1; Sc1P=0; Sc2P=0;
            a = a+0.000001; %pause(Tc/4);
        end
    end     
end
if(Sector5)
    if(rgn3)
        while(a<exttime+Tc/4)
            Sa1=0; Sa2=1; Sa1P=1; Sa2P=0;
            Sb1=0; Sb2=1; Sb1P=1; Sb2P=0;
            Sc1=1; Sc2=1; Sc1P=0; Sc2P=0;
            a = a+0.000001; %pause(Tc/4);
        end
        while(a<exttime+Tb/2)
            Sa1=0; Sa2=1; Sa1P=1; Sa2P=0;
            Sb1=0; Sb2=0; Sb1P=1; Sb2P=1;
            Sc1=1; Sc2=1; Sc1P=0; Sc2P=0;
            a = a+0.000001; %pause(Tb/2); 
        end
        while(a<exttime+Ta/2)
            Sa1=0; Sa2=0; Sa1P=1; Sa2P=1;
            Sb1=0; Sb2=0; Sb1P=1; Sb2P=1;
            Sc1=1; Sc2=1; Sc1P=0; Sc2P=0;
            a = a+0.000001; %pause(Ta/2); 
        end
        while(a<exttime+Tc/2)
            Sa1=0; Sa2=0; Sa1P=1; Sa2P=1;
            Sb1=0; Sb2=0; Sb1P=1; Sb2P=1;
            Sc1=0; Sc2=1; Sc1P=1; Sc2P=0;
            a = a+0.000001; %pause(Tc/2);
        end
        while(a<exttime+Ta/2)
            Sa1=0; Sa2=0; Sa1P=1; Sa2P=1;
            Sb1=0; Sb2=0; Sb1P=1; Sb2P=1;
            Sc1=1; Sc2=1; Sc1P=0; Sc2P=0;
            a = a+0.000001; %pause(Ta/2); 
        end
        while(a<exttime+Tb/2)
            Sa1=0; Sa2=1; Sa1P=1; Sa2P=0;
            Sb1=0; Sb2=0; Sb1P=1; Sb2P=1;
            Sc1=1; Sc2=1; Sc1P=0; Sc2P=0;
            a = a+0.000001; %pause(Tb/2); 
        end
        while(a<exttime+Tc/4)
            Sa1=0; Sa2=1; Sa1P=1; Sa2P=0;
            Sb1=0; Sb2=1; Sb1P=1; Sb2P=0;
            Sc1=1; Sc2=1; Sc1P=0; Sc2P=0;
            a = a+0.000001; %pause(Tc/4);
        end
    end
        if(rgn2a)
            while(a<exttime+Tc/4)
                Sa1=0; Sa2=1; Sa1P=1; Sa2P=0;
                Sb1=0; Sb2=1; Sb1P=1; Sb2P=0;
                Sc1=1; Sc2=1; Sc1P=0; Sc2P=0;
                a = a+0.000001; %pause(Tc/4);
            end
            while(a<exttime+Tb/2)
                Sa1=0; Sa2=1; Sa1P=1; Sa2P=0;
                Sb1=0; Sb2=0; Sb1P=1; Sb2P=1;
                Sc1=1; Sc2=1; Sc1P=0; Sc2P=0;
                a = a+0.000001; %pause(Tb/2); 
            end
            while(a<exttime+Ta/2)
                Sa1=0; Sa2=1; Sa1P=1; Sa2P=0;
                Sb1=0; Sb2=0; Sb1P=1; Sb2P=1;
                Sc1=0; Sc2=1; Sc1P=1; Sc2P=0;        
                a = a+0.000001; %pause(Ta/2); 
            end
            while(a<exttime+Tc/2)
                Sa1=0; Sa2=0; Sa1P=1; Sa2P=1;
                Sb1=0; Sb2=0; Sb1P=1; Sb2P=1;
                Sc1=0; Sc2=1; Sc1P=1; Sc2P=0;
                a = a+0.000001; %pause(Tc/2);
            end
            while(a<exttime+Ta/2)
                Sa1=0; Sa2=1; Sa1P=1; Sa2P=0;
                Sb1=0; Sb2=0; Sb1P=1; Sb2P=1;
                Sc1=0; Sc2=1; Sc1P=1; Sc2P=0;        
                a = a+0.000001; %pause(Ta/2); 
            end
            while(a<exttime+Tb/2)
                Sa1=0; Sa2=1; Sa1P=1; Sa2P=0;
                Sb1=0; Sb2=0; Sb1P=1; Sb2P=1;
                Sc1=1; Sc2=1; Sc1P=0; Sc2P=0;
                a = a+0.000001; %pause(Tb/2); 
            end
            while(a<exttime+Tc/4)
                Sa1=0; Sa2=1; Sa1P=1; Sa2P=0;
                Sb1=0; Sb2=1; Sb1P=1; Sb2P=0;
                Sc1=1; Sc2=1; Sc1P=0; Sc2P=0;
                a = a+0.000001;%pause(Tc/4);
            end
        end
        if(rgn2b)
            while(a<exttime+Tc/4)
                Sa1=1; Sa2=1; Sa1P=0; Sa2P=0;
                Sb1=0; Sb2=1; Sb1P=1; Sb2P=0;
                Sc1=1; Sc2=1; Sc1P=0; Sc2P=0;
                a = a+0.000001; %pause(Tc/4);
            end
            while(a<exttime+Tb/2)
                Sa1=0; Sa2=1; Sa1P=1; Sa2P=0;
                Sb1=0; Sb2=1; Sb1P=1; Sb2P=0;
                Sc1=1; Sc2=1; Sc1P=0; Sc2P=0;
                a = a+0.000001; %pause(Tb/2); 
            end
            while(a<exttime+Ta/2)
                Sa1=0; Sa2=1; Sa1P=1; Sa2P=0;
                Sb1=0; Sb2=0; Sb1P=1; Sb2P=1;
                Sc1=1; Sc2=1; Sc1P=0; Sc2P=0;
                a = a+0.000001; %pause(Ta/2); 
            end
            while(a<exttime+Tc/2)
                Sa1=0; Sa2=1; Sa1P=1; Sa2P=0;
                Sb1=0; Sb2=0; Sb1P=1; Sb2P=1;
                Sc1=0; Sc2=1; Sc1P=1; Sc2P=0;
                a = a+0.000001; %pause(Tc/2);
            end
            while(a<exttime+Ta/2)
                Sa1=0; Sa2=1; Sa1P=1; Sa2P=0;
                Sb1=0; Sb2=0; Sb1P=1; Sb2P=1;
                Sc1=1; Sc2=1; Sc1P=0; Sc2P=0;
                a = a+0.000001; %pause(Ta/2); 
            end
            while(a<exttime+Tb/2)
                Sa1=0; Sa2=1; Sa1P=1; Sa2P=0;
                Sb1=0; Sb2=1; Sb1P=1; Sb2P=0;
                Sc1=1; Sc2=1; Sc1P=0; Sc2P=0;
                a = a+0.000001; %pause(Tb/2); 
            end
            while(a<exttime+Tc/4)
                Sa1=1; Sa2=1; Sa1P=0; Sa2P=0;
                Sb1=0; Sb2=1; Sb1P=1; Sb2P=0;
                Sc1=1; Sc2=1; Sc1P=0; Sc2P=0;
                a = a+0.000001; %pause(Tc/4);               
            end
        end
    if(rgn4)
        while(a<exttime+Tc/4)
            Sa1=1; Sa2=1; Sa1P=0; Sa2P=0; 
            Sb1=0; Sb2=1; Sb1P=1; Sb2P=0;
            Sc1=1; Sc2=1; Sc1P=0; Sc2P=0;
            a = a+0.000001; %pause(Tc/4);
        end
        while(a<exttime+Tb/2)
            Sa1=1; Sa2=1; Sa1P=0; Sa2P=0;
            Sb1=0; Sb2=0; Sb1P=1; Sb2P=1;
            Sc1=1; Sc2=1; Sc1P=0; Sc2P=0;
            a = a+0.000001; %pause(Tb/2); 
        end
        while(a<exttime+Ta/2)
            Sa1=0; Sa2=1; Sa1P=1; Sa2P=0;
            Sb1=0; Sb2=0; Sb1P=1; Sb2P=1;
            Sc1=1; Sc2=1; Sc1P=0; Sc2P=0;
            a = a+0.000001; %pause(Ta/2); 
        end
        while(a<exttime+Tc/2)
            Sa1=0; Sa2=1; Sa1P=1; Sa2P=0;
            Sb1=0; Sb2=0; Sb1P=1; Sb2P=1;
            Sc1=0; Sc2=1; Sc1P=1; Sc2P=0;
            a = a+0.000001; %pause(Tc/2);
        end
        while(a<exttime+Ta/2)
            Sa1=0; Sa2=1; Sa1P=1; Sa2P=0;
            Sb1=0; Sb2=0; Sb1P=1; Sb2P=1;
            Sc1=1; Sc2=1; Sc1P=0; Sc2P=0;
            a = a+0.000001; %pause(Ta/2); 
        end
        while(a<exttime+Tb/2)
            Sa1=1; Sa2=1; Sa1P=0; Sa2P=0;
            Sb1=0; Sb2=0; Sb1P=1; Sb2P=1;
            Sc1=1; Sc2=1; Sc1P=0; Sc2P=0;
            a = a+0.000001; %pause(Tb/2); 
        end
        while(a<exttime+Tc/4)
            Sa1=1; Sa2=1; Sa1P=0; Sa2P=0; 
            Sb1=0; Sb2=1; Sb1P=1; Sb2P=0;
            Sc1=1; Sc2=1; Sc1P=0; Sc2P=0;
            a = a+0.000001; %pause(Tc/4);
        end
    end
    
end
if(Sector6)
    if(rgn3)
        while(a<exttime+Tc/4)
            Sa1=1; Sa2=1; Sa1P=0; Sa2P=0;
            Sb1=0; Sb2=1; Sb1P=1; Sb2P=0;
            Sc1=1; Sc2=1; Sc1P=0; Sc2P=0;
            a = a+0.000001; %pause(Tc/4);
        end
        while(a<exttime+Tb/2)
            Sa1=1; Sa2=1; Sa1P=0; Sa2P=0;
            Sb1=0; Sb2=0; Sb1P=1; Sb2P=1;
            Sc1=1; Sc2=1; Sc1P=0; Sc2P=0;
            a = a+0.000001; %pause(Tb/2); 
        end
        while(a<exttime+Ta/2)
            Sa1=1; Sa2=1; Sa1P=0; Sa2P=0;
            Sb1=0; Sb2=0; Sb1P=1; Sb2P=1;
            Sc1=0; Sc2=1; Sc1P=1; Sc2P=0;
            a = a+0.000001; %pause(Ta/2); 
        end
        while(a<exttime+Tc/2)
            Sa1=0; Sa2=1; Sa1P=1; Sa2P=0;
            Sb1=0; Sb2=0; Sb1P=1; Sb2P=1;
            Sc1=0; Sc2=1; Sc1P=1; Sc2P=0;
            a = a+0.000001; %pause(Tc/2);
        end
        while(a<exttime+Ta/2)
            Sa1=1; Sa2=1; Sa1P=0; Sa2P=0;
            Sb1=0; Sb2=0; Sb1P=1; Sb2P=1;
            Sc1=0; Sc2=1; Sc1P=1; Sc2P=0;
            a = a+0.000001; %pause(Ta/2); 
        end
        while(a<exttime+Tb/2)
            Sa1=1; Sa2=1; Sa1P=0; Sa2P=0;
            Sb1=0; Sb2=0; Sb1P=1; Sb2P=1;
            Sc1=1; Sc2=1; Sc1P=0; Sc2P=0;
            a = a+0.000001; %pause(Tb/2); 
        end
        while(a<exttime+Tc/4)
            Sa1=1; Sa2=1; Sa1P=0; Sa2P=0;
            Sb1=0; Sb2=1; Sb1P=1; Sb2P=0;
            Sc1=1; Sc2=1; Sc1P=0; Sc2P=0;
            a = a+0.000001; %pause(Tc/4);
        end
    end
        if(rgn2a)
            while(a<exttime+Tc/4)
                Sa1=1; Sa2=1; Sa1P=0; Sa2P=0;
                Sb1=0; Sb2=1; Sb1P=1; Sb2P=0;
                Sc1=1; Sc2=1; Sc1P=0; Sc2P=0;
                a = a+0.000001; %pause(Tc/4);
            end
            while(a<exttime+Tb/2)
                Sa1=1; Sa2=1; Sa1P=0; Sa2P=0;
                Sb1=0; Sb2=1; Sb1P=1; Sb2P=0;
                Sc1=0; Sc2=1; Sc1P=1; Sc2P=0;
                a = a+0.000001; %pause(Tb/2); 
            end
            while(a<exttime+Ta/2)
                Sa1=1; Sa2=1; Sa1P=0; Sa2P=0;
                Sb1=0; Sb2=0; Sb1P=1; Sb2P=1;
                Sc1=0; Sc2=1; Sc1P=1; Sc2P=0;
                a = a+0.000001; %pause(Ta/2); 
            end
            while(a<exttime+Tc/2)
                Sa1=0; Sa2=1; Sa1P=1; Sa2P=0;
                Sb1=0; Sb2=0; Sb1P=1; Sb2P=1;
                Sc1=0; Sc2=1; Sc1P=1; Sc2P=0;
                a = a+0.000001; %pause(Tc/2);
            end
            while(a<exttime+Ta/2)
                Sa1=1; Sa2=1; Sa1P=0; Sa2P=0;
                Sb1=0; Sb2=0; Sb1P=1; Sb2P=1;
                Sc1=0; Sc2=1; Sc1P=1; Sc2P=0;
                a = a+0.000001; %pause(Ta/2); 
            end
            while(a<exttime+Tb/2)
                Sa1=1; Sa2=1; Sa1P=0; Sa2P=0;
                Sb1=0; Sb2=1; Sb1P=1; Sb2P=0;
                Sc1=0; Sc2=1; Sc1P=1; Sc2P=0;
                a = a+0.000001; %pause(Tb/2);  
            end
            while(a<exttime+Tc/4)
                Sa1=1; Sa2=1; Sa1P=0; Sa2P=0;
                Sb1=0; Sb2=1; Sb1P=1; Sb2P=0;
                Sc1=1; Sc2=1; Sc1P=0; Sc2P=0;
                a = a+0.000001; %pause(Tc/4);
            end
        end
        if(rgn2b)
            while(a<exttime+Tc/4)
                Sa1=1; Sa2=1; Sa1P=0; Sa2P=0;
                Sb1=0; Sb2=1; Sb1P=1; Sb2P=0;
                Sc1=0; Sc2=1; Sc1P=1; Sc2P=0;
                a = a+0.000001; %pause(Tc/4);
            end
            while(a<exttime+Tb/2)
                Sa1=1; Sa2=1; Sa1P=0; Sa2P=0;
                Sb1=0; Sb2=0; Sb1P=1; Sb2P=1;
                Sc1=0; Sc2=1; Sc1P=1; Sc2P=0;
                a = a+0.000001; %pause(Tb/2); 
            end
            while(a<exttime+Ta/2)
                Sa1=0; Sa2=1; Sa1P=1; Sa2P=0;
                Sb1=0; Sb2=0; Sb1P=1; Sb2P=1;
                Sc1=0; Sc2=1; Sc1P=1; Sc2P=0;
                a = a+0.000001; %pause(Ta/2); 
            end
            while(a<exttime+Tc/2)
                Sa1=0; Sa2=1; Sa1P=1; Sa2P=0;
                Sb1=0; Sb2=0; Sb1P=1; Sb2P=1;
                Sc1=0; Sc2=0; Sc1P=1; Sc2P=1;
                a = a+0.000001; %pause(Tc/2);
            end
            while(a<exttime+Ta/2)
                Sa1=0; Sa2=1; Sa1P=1; Sa2P=0;
                Sb1=0; Sb2=0; Sb1P=1; Sb2P=1;
                Sc1=0; Sc2=1; Sc1P=1; Sc2P=0;
                a = a+0.000001; %pause(Ta/2); 
            end
            while(a<exttime+Tb/2)
                Sa1=1; Sa2=1; Sa1P=0; Sa2P=0;
                Sb1=0; Sb2=0; Sb1P=1; Sb2P=1;
                Sc1=0; Sc2=1; Sc1P=1; Sc2P=0;
                a = a+0.000001; %pause(Tb/2); 
            end
            while(a<exttime+Tc/4)
                Sa1=1; Sa2=1; Sa1P=0; Sa2P=0;
                Sb1=0; Sb2=1; Sb1P=1; Sb2P=0;
                Sc1=0; Sc2=1; Sc1P=1; Sc2P=0;
                a = a+0.000001; %pause(Tc/4);
            end
        end
    if(rgn4)
        while(a<exttime+Tc/4)
            Sa1=1; Sa2=1; Sa1P=0; Sa2P=0;
            Sb1=0; Sb2=1; Sb1P=1; Sb2P=0;
            Sc1=0; Sc2=1; Sc1P=1; Sc2P=0;
            a = a+0.000001; %pause(Tc/4);
        end
        while(a<exttime+Tb/2)
            Sa1=1; Sa2=1; Sa1P=0; Sa2P=0;
            Sb1=0; Sb2=0; Sb1P=1; Sb2P=1;
            Sc1=0; Sc2=1; Sc1P=1; Sc2P=0;
            a = a+0.000001; %pause(Tb/2); 
        end
        while(a<exttime+Ta/2)
            Sa1=1; Sa2=1; Sa1P=0; Sa2P=0;
            Sb1=0; Sb2=0; Sb1P=1; Sb2P=1;
            Sc1=0; Sc2=0; Sc1P=1; Sc2P=1;
            a = a+0.000001; %pause(Ta/2); 
        end
        while(a<exttime+Tc/2)
            Sa1=0; Sa2=1; Sa1P=1; Sa2P=0;
            Sb1=0; Sb2=0; Sb1P=1; Sb2P=1;
            Sc1=0; Sc2=0; Sc1P=1; Sc2P=1;
            a = a+0.000001; %pause(Tc/2);
        end
        while(a<exttime+Ta/2)
            Sa1=1; Sa2=1; Sa1P=0; Sa2P=0;
            Sb1=0; Sb2=0; Sb1P=1; Sb2P=1;
            Sc1=0; Sc2=0; Sc1P=1; Sc2P=1;
            a = a+0.000001; %pause(Ta/2); 
        end
        while(a<exttime+Tb/2)
            Sa1=1; Sa2=1; Sa1P=0; Sa2P=0;
            Sb1=0; Sb2=0; Sb1P=1; Sb2P=1;
            Sc1=0; Sc2=1; Sc1P=1; Sc2P=0;
            a = a+0.000001; %pause(Tb/2);  
        end
        while(a<exttime+Tc/4)
            Sa1=1; Sa2=1; Sa1P=0; Sa2P=0;
            Sb1=0; Sb2=1; Sb1P=1; Sb2P=0;
            Sc1=0; Sc2=1; Sc1P=1; Sc2P=0;
            a = a+0.000001; %pause(Tc/4);
        end
    end
end




%% test
%output = Ts/(Ta+Tb+Tc);
%% duty cycles 
%da = Ta/Ts;
%db = Tb/Ts;
%dc = Tc/Ts;
